simulink model "ModeAdjust"  (R2018b)
settings: Solver=FixedStepDiscrete  StartTime=0.0  StopTime=inf  FixedStep=0.01  RelTol=1e-3
undefined symbols (not defined in the file or in its folder): IfKeSMSbSeatMovBkRclnEnable_Val, IfKeSMSbSeatMovFrwdBkwdEnable_Val, IfKeSMSbSeatMovFtrstEnable_Val, IfKeSMSbSeatMovHdrstFrwdBkwdEnable_Val, IfKeSMSbSeatMovHdUpwdDnwdEnable_Val, IfKeSMSbSeatMovLgrstEnable_Val, IfKeSMSbSeatMovLtwdRtwdEnable_Val, IfVeSMSeStNumConfig, KeSMSbArmscreenMovEnable_Val, KeSMSbSeatMovLgrstExpdEnable_Val, KeSMSuFirstRwStBackPosDelta_Val, KeSMSuFirstRwStBackPosTolr_Val, KeSMSuFirstRwStCushFrntPosDelta_Val, KeSMSuFirstRwStCushFrntPosTolr_Val, KeSMSuFirstRwStCushRePosDelta_Val, KeSMSuFirstRwStCushRePosTolr_Val, KeSMSuFirstRwStFootrestPosDelta_Val, KeSMSuFirstRwStFootrestPosTolr_Val, KeSMSuFirstRwStFwdBkwdPosDelta_Val, KeSMSuFirstRwStFwdBkwdPosTolr_Val, KeSMSuMdMotFinshdTm_Val, KeSMSuMdRetryTm1_Val, KeSMSuModeReqDurgTm_Val, KeSMSuSecRwStArmTochPosDelta_Val, KeSMSuSecRwStArmTochPosTolr_Val, KeSMSuSecRwStBackPosDelta_Val, KeSMSuSecRwStBackPosTolr_Val, KeSMSuSecRwStFtrstUpwdDnwdPosDelta_Val, KeSMSuSecRwStFtrstUpwdDnwdPosTolr_Val, KeSMSuSecRwStFwdBkwdPosDelta_Val, KeSMSuSecRwStFwdBkwdPosTolr_Val, KeSMSuSecRwStHeadrestFwdBkwdPosDelta_Val, KeSMSuSecRwStHeadrestFwdBkwdPosTolr_Val, KeSMSuSecRwStHeadrestUpwdDwnwdPosDelta_Val, KeSMSuSecRwStHeadrestUpwdDwnwdPosTolr_Val, KeSMSuSecRwStLegrestInOutPosDelta_Val, KeSMSuSecRwStLegrestInOutPosTolr_Val, KeSMSuSecRwStLegrestUpwdDwnwdPosDelta_Val, KeSMSuSecRwStLegrestUpwdDwnwdPosTolr_Val, KeSMSuSecRwStLwdRwdPosDelta_Val, KeSMSuSecRwStLwdRwdPosTolr_Val, KeSMSuSecRwStVIPFtrstRefAngle_Val, KeSMSuThirdRwStFwdBkwdPosDelta_Val, KeSMSuThirdRwStFwdBkwdPosTolr_Val, KeSMSuThrdRwCushFoldPosDelta_Val, KeSMSuThrdRwCushFoldPosTolr_Val, KeSMSuThrdRwStBackPosDelta_Val, KeSMSuThrdRwStBackPosTolr_Val, KeSMSw4SLegrstCloseMdSecRwLtStFtrstUpwdDnwdPos_Val, KeSMSw4SLegrstCloseMdSecRwLtStFtrstUpwdDnwdPosMax_Val, KeSMSw4SLegrstCloseMdSecRwLtStFtrstUpwdDnwdPosMin_Val, KeSMSw4SLegrstCloseMdSecRwLtStLgrstOtwdInwdPos_Val, KeSMSw4SLegrstCloseMdSecRwLtStLgrstOtwdInwdPosMax_Val, KeSMSw4SLegrstCloseMdSecRwLtStLgrstOtwdInwdPosMin_Val, KeSMSw4SLegrstCloseMdSecRwLtStLgrstUpwdDnwdPos_Val, KeSMSw4SLegrstCloseMdSecRwLtStLgrstUpwdDnwdPosMax_Val, KeSMSw4SLegrstCloseMdSecRwLtStLgrstUpwdDnwdPosMin_Val, KeSMSw4SLegrstCloseMdSecRwRtStFtrstUpwdDnwdPos_Val, KeSMSw4SLegrstCloseMdSecRwRtStFtrstUpwdDnwdPosMax_Val, KeSMSw4SLegrstCloseMdSecRwRtStFtrstUpwdDnwdPosMin_Val ... (+1138)
libraries: Lib x401
(part 11 of 35)

== system ModeAdjust/ModeAdjustRunnable_sys/ModeAdjust/VIPR4s ==
  SecRwLtStsPoss : Inport
  SecRwLtStPossV : Inport  Port=2
  SecRwRtStChldLkRsp_L : Inport  Port=3
  Recovery_Mod_Left : Inport  Port=4
  ModeStCalib : Inport  Port=5
  StConfig : Inport  Port=6
  SecRwLtStsPoss4s : Inport  Port=7
  SecRwLtStPossV4s : Inport  Port=8
  StConfig4s : Inport  Port=9
  isRtVipArrivedAtTargetPos : Inport  Port=10
  Calib_VIP4sRAdpt : Inport  Port=11
  Enable : EnablePort  StatesWhenEnabling=reset
  Bus Creator1 : BusCreator  Inputs=2
  Bus Selector : BusSelector  OutputSignals=Calib_Drv,Calib_Pass,Calib_2L,Calib_2R,Calib_3L,Calib_3R,Calib_2L4s,Calib_2R4s
  Bus Selector1 : BusSelector  OutputSignals=DrvStConfig,PassStConfig,SecRwLtStConfig,SecRwRtStConfig,ThdRwLtStConfig,ThdRwRtStConfig
  Bus Selector2 : BusSelector  OutputSignals=SecRwLtStConfig,SecRwRtStConfig
  Bus Selector3 : BusSelector  OutputSignals=IfVeSMSuSecRwRtStBkReclnUpwdDnwdPos_Val_read,IfVeSMSuSecRwRtStFrwdBkwdPos_Val_read,IfVeSMSuSecRwRtStHPassStUpwdDnwdPos_Val_read,IfVeSMSuSecRwRtStLgrstUpwdDnwdPos_Val_read,IfVeSMSuSecRwRtStLtwdRtwdPos_Val_read,SecRwRtStArmScrnPos_Val_read
  Bus Selector4 : BusSelector  OutputSignals=IfVeSMSuSecRwRtStBkReclnUpwdDnwdPosV_Val_read,IfVeSMSuSecRwRtStFrwdBkwdPosV_Val_read,IfVeSMSuSecRwRtStHPassStUpwdDnwdPosV_Val_read,IfVeSMSuSecRwRtStLgrstUpwdDnwdPosV_Val_read,IfVeSMSuSecRwRtStLtwdRtwdPosV_Val_read,SecRwRtStArmScrnPosV_Val_read
  Bus Selector5 : BusSelector  OutputSignals=IfVeSMSuSecRwRtStLgrstOtwdInwdPos_Val_read,IfVeSMSuRrRtStFtUpwdDnwdPos_Val_read,IfVeSMSuSecRwRtStHdrstFrwdBkwdPos_Val_read
  Bus Selector6 : BusSelector  OutputSignals=IfVeSMSuSecRwRtStLgrstOtwdInwdPosV_Val_read,IfVeSMSuRrRtStFtUpwdDnwdPosV_Val_read
  Bus Selector7 : BusSelector  OutputSignals=VipRSecRwRtSt.HdrstFrwdBkwdnwdPos,VipRSecRwRtSt.FtrstUpwdDnwdPos
  Chart : Stateflow chart  TreatAsAtomicUnit=on
  Chart1 : Stateflow chart  TreatAsAtomicUnit=on
  Logical Operator : Logic  Inputs=4  AllPortsSameDT=off  OutDataTypeStr=boolean
  Logical Operator1 : Logic  Inputs=3  AllPortsSameDT=off  OutDataTypeStr=boolean
  Logical Operator2 : Logic  AllPortsSameDT=off  OutDataTypeStr=boolean
  Logical Operator3 : Logic  AllPortsSameDT=off  OutDataTypeStr=boolean
  Logical Operator4 : Logic  Operator=NOT  AllPortsSameDT=off  OutDataTypeStr=boolean
  Logical Operator5 : Logic  AllPortsSameDT=off  OutDataTypeStr=boolean
  Logical Operator{6..9} (4 alike) : Logic  Operator=OR  AllPortsSameDT=off  OutDataTypeStr=boolean
  PA_KeSMSw4SSecRwRtStLgrstUpwdDnwdOpenPos1_Val : Constant  Value=KeSMSw4SSecRwRtStLgrstUpwdDnwdOpenPos1_Val
  R2Lt : Subsystem
  Relational Operator : RelationalOperator  OutDataTypeStr=boolean  RndMeth=Simplest
  Relational Operator1 : RelationalOperator  Operator=<  OutDataTypeStr=boolean  RndMeth=Simplest
  Relational Operator2 : RelationalOperator  Operator=<  OutDataTypeStr=boolean  RndMeth=Simplest
  Unit Delay1 : UnitDelay  SampleTime=-1
  Unit Delay3 : UnitDelay  SampleTime=-1
  Unit Delay4 : UnitDelay  SampleTime=-1
  VIP_TrigJudg : Lib/VIP_TrigJudg  SystemSampleTime=-1
  R2Lt_TrgtPoss : Outport  VectorParamsAs1DForOutWhenUnconnected=on
  IfVeSMSuSecRwLtStRclCmdSrv_Val_writeRec : Outport  Port=2
  isAcsMdFeedBackNew_LyL : Outport  Port=3
  R2Lt_TrgtPoss_2 : Outport  Port=4  VectorParamsAs1DForOutWhenUnconnected=on
  wires:
  Unit Delay4/1 -> Logical Operator3/2
  Relational Operator/1 -> Unit Delay3/1
  [lgrstStep2_done] -> Logical Operator2/2
  Logical Operator2/1 -> Unit Delay1/1
  [SecRwLtStLgrstUpwdDnwdPos] -> Relational Operator/1
  [lgrstStep3_done] -> Logical Operator3/1
  Unit Delay3/1 -> Logical Operator2/1
  [lgrstStep2_Chk] -> Unit Delay4/1
  [OpenPos1] -> Relational Operator/2
  R2Lt/4(IfVeSMSuSecRwLtStRclCmdSrv_Val_writeRaw) -> [IfVeSMSuSecRwLtStRclCmdSrv_Val_writeRaw]
  [IfVeSMSuSecRwLtStRclCmdSrv_Val_writeRaw] -> Chart1/2(IfVeSMSuSecRwLtStRclCmdSrv_Val_writeRaw)
  Recovery_Mod_Left/1 -> [Recovery_Mod_Left]
  R2Lt/1(R2Lt_BkHd_Ini) -> [R2LtST_BkHd_ini]
  [Step1_En] -> R2Lt/2(Step1En)
  VIP_TrigJudg/1 -> [EZE_TrigL]
  [EZE_TrigL] -> R2Lt/1(Mode_Trig)
  R2Lt/3(R2Lt_TrgtPoss) -> R2Lt_TrgtPoss/1
  SecRwLtStsPoss/1 -> [Pos], R2Lt/3(SecRwLtStsPoss)
  SecRwLtStPossV/1 -> [PosV], R2Lt/4(SecRwLtStPossV)
  SecRwRtStChldLkRsp_L/1 -> R2Lt/5(SecRwRtStChldLkRsp_L)
  R2Lt/2(R2Lt_BkHd_done) -> [R2LtST_BkHd_done]
  [R2LtST_BkHd_ini] -> Chart/1(R2Lt_ini)
  [R2LtST_BkHd_done] -> Chart/2(R2Lt_done)
  [Recv_L_DoneOK] -> Chart1/3(Md_L_DoneOkRaw)
  [Recv_L_DoneFailed] -> Chart1/4(Md_L_DoneFailedRaw)
  Chart1/2(Md_L_DoneOk) -> [Ly_L_DoneOK]
  Chart1/3(Md_L_DoneFailed) -> [Ly_L_DoneFailed]
  Chart1/1(IfVeSMSuSecRwLtStRclCmdSrv_Val_write) -> IfVeSMSuSecRwLtStRclCmdSrv_Val_writeRec/1  "IfVeSMSuSecRwLtStRclCmdSrv_Val_write"
  Bus Selector/2 -> [ModeStCalib_Pass]  "<Calib_Pass>"
  Bus Selector/5 -> [ModeStCalib_3L]  "<Calib_3L>"
  Bus Selector/3 -> [ModeStCalib_2L]  "<Calib_2L>"
  Bus Selector/1 -> [ModeStCalib_Drv]  "<Calib_Drv>"
  Bus Selector/6 -> [ModeStCalib_3R]  "<Calib_3R>"
  Bus Selector/4 -> [ModeStCalib_2R]  "<Calib_2R>"
  ModeStCalib/1 -> Bus Selector/1
  [ModeStCalib_2R4s] -> R2Lt/6(ModeStCalib_2L)
  [Recovery_Mod_Left] -> VIP_TrigJudg/1
  Bus Creator1/1 -> isAcsMdFeedBackNew_LyL/1
  [Ly_L_DoneOK] -> Bus Creator1/1  "isRtVipDoneOK"
  [Ly_L_DoneFailed] -> Bus Creator1/2  "isRtVipDoneFailed"
  Bus Selector1/6 -> [ThdRwRtStConfig]  "<ThdRwRtStConfig>"
  Bus Selector1/1 -> [DrvStConfig]  "<DrvStConfig>"
  Bus Selector1/3 -> [SecRwLtStConfig]  "<SecRwLtStConfig>"
  Bus Selector1/4 -> [SecRwRtStConfig]  "<SecRwRtStConfig>"
  StConfig/1 -> Bus Selector1/1
  Bus Selector1/2 -> [PassStConfig]  "<PassStConfig>"
  Bus Selector1/5 -> [ThdRwLtStConfig]  "<ThdRwLtStConfig>"
  [SecRwLtStConfig] -> R2Lt/7(StConfig)
  Bus Selector/8 -> [ModeStCalib_2R4s]  "<Calib_2R4s>"
  Bus Selector/7 -> [ModeStCalib_2L4s]  "<Calib_2L4s>"
  SecRwLtStsPoss4s/1 -> [Pos4s], R2Lt/8(SecRwLtStsPoss4s)
  SecRwLtStPossV4s/1 -> [PosV4s], R2Lt/9(SecRwLtStPossV4s)
  StConfig4s/1 -> Bus Selector2/1
  Bus Selector2/1 -> [SecRwLtStConfig4s]  "<SecRwLtStConfig>"
  Bus Selector2/2 -> [SecRwRtStConfig4s]  "<SecRwRtStConfig>"
  [SecRwLtStConfig4s] -> R2Lt/10(StConfig4s)
  [PosV] -> Bus Selector4/1
  Bus Selector4/6 -> [R2LtStArmScrnPosV]  "<SecRwRtStArmScrnPosV_Val_read>"
  Bus Selector3/6 -> [R2LtStArmScrnPos]  "<SecRwRtStArmScrnPos_Val_read>"
  Bus Selector4/5 -> [SecRwLtStLtwdRtwdPosV]  "<IfVeSMSuSecRwRtStLtwdRtwdPosV_Val_read>"
  Bus Selector3/4 -> [SecRwLtStLgrstUpwdDnwdPos]  "<IfVeSMSuSecRwRtStLgrstUpwdDnwdPos_Val_read>"
  Bus Selector3/1 -> [SecRwLtStBkReclnUpwdDnwdPos]  "<IfVeSMSuSecRwRtStBkReclnUpwdDnwdPos_Val_read>"
  Bus Selector3/2 -> [SecRwLtStFrwdBkwdPos]  "<IfVeSMSuSecRwRtStFrwdBkwdPos_Val_read>"
  Bus Selector4/2 -> [SecRwLtStFrwdBkwdPosV]  "<IfVeSMSuSecRwRtStFrwdBkwdPosV_Val_read>"
  Bus Selector4/4 -> [SecRwLtStLgrstUpwdDnwdPosV]  "<IfVeSMSuSecRwRtStLgrstUpwdDnwdPosV_Val_read>"
  Bus Selector3/3 -> [SecRwLtStHPassStUpwdDnwdPos]  "<IfVeSMSuSecRwRtStHPassStUpwdDnwdPos_Val_read>"
  [Pos] -> Bus Selector3/1
  Bus Selector3/5 -> [SecRwLtStLtwdRtwdPos]  "<IfVeSMSuSecRwRtStLtwdRtwdPos_Val_read>"
  Bus Selector4/3 -> [SecRwLtStHPassStUpwdDnwdPosV]  "<IfVeSMSuSecRwRtStHPassStUpwdDnwdPosV_Val_read>"
  Bus Selector4/1 -> [SecRwLtStBkReclnUpwdDnwdPosV]  "<IfVeSMSuSecRwRtStBkReclnUpwdDnwdPosV_Val_read>"
  Bus Selector6/1 -> [SecRwLtStLgrstOtwdInwdPosV]  "<IfVeSMSuSecRwRtStLgrstOtwdInwdPosV_Val_read>"
  [Pos4s] -> Bus Selector5/1
  Bus Selector6/2 -> [RrLtStFtUpwdDnwdPosV]  "<IfVeSMSuRrRtStFtUpwdDnwdPosV_Val_read>"
  [PosV4s] -> Bus Selector6/1
  Bus Selector5/1 -> [SecRwLtStLgrstOtwdInwdPos]  "<IfVeSMSuSecRwRtStLgrstOtwdInwdPos_Val_read>"
  Bus Selector5/2 -> [RrLtStFtUpwdDnwdPos]  "<IfVeSMSuRrRtStFtUpwdDnwdPos_Val_read>"
  [SecRwLtStLgrstUpwdDnwdPos] -> Chart/3(pos)
  [StepEn_LgrstStep1] -> R2Lt/11(StepEn_LgrstStep1)
  [StepEn_LgrstStep2] -> R2Lt/12(StepEn_LgrstStep2)
  [StepEn_LgrstStep3] -> R2Lt/13(StepEn_LgrstStep3)
  R2Lt/5(lgrstStep1_ini) -> [lgrstStep1_ini]
  R2Lt/7(lgrstStep3_ini) -> [lgrstStep3_ini]
  R2Lt/6(lgrstStep2_ini) -> [lgrstStep2_ini]
  R2Lt/8(lgrstStep1_done) -> [lgrstStep1_done]
  R2Lt/10(lgrstStep3_done) -> [lgrstStep3_done]
  R2Lt/9(lgrstStep2_done) -> [lgrstStep2_done]
  [lgrstStep1_done] -> Chart/5(Step1done)
  [lgrstStep1_ini] -> Chart/8(Step1_ini)
  [lgrstStep2_ini] -> Chart/9(Step2_ini)
  [lgrstStep3_ini] -> Chart/10(Step3_ini)
  PA_KeSMSw4SSecRwRtStLgrstUpwdDnwdOpenPos1_Val/1 -> [OpenPos1]
  [OpenPos1] -> Chart/4(openpos1)
  Logical Operator3/1 -> Chart/7(Step3done), [lgrstStep3_Chk]
  Unit Delay1/1 -> Chart/6(Step2done), [lgrstStep2_Chk]
  R2Lt/11(R2Lt_TrgtPoss_2) -> R2Lt_TrgtPoss_2/1
  Logical Operator4/1 -> [Recv_L_DoneFailed]
  isRtVipArrivedAtTargetPos/1 -> [Recv_L_DoneOK], Logical Operator4/1
  [HdUp_Done] -> Logical Operator/3
  [HFwd_Done] -> Logical Operator/4
  [failflg] -> Logical Operator6/2
  Logical Operator1/1 -> Logical Operator6/1
  [R2LtST_BkHd_done] -> Logical Operator/2
  Logical Operator/1 -> Chart1/1(Left_Done)
  Logical Operator6/1 -> Logical Operator/1
  Chart/1(R2Lt_En) -> [Step1_En]
  [HdUp_Done] -> Chart/12(HdUp_Done)
  Chart/7(failflg) -> [failflg]
  Chart/5(HdUp_En) -> [HdUp_En]
  [HFwd_Done] -> Chart/13(HdFwd_Done)
  Chart/2(StepEn_LgrstStep1) -> [StepEn_LgrstStep1]
  Bus Selector7/1 -> Relational Operator1/2  "<HdrstFrwdBkwdnwdPos>"
  [SecRwLtStHdrstFrwdBkwdPos] -> Relational Operator1/1
  Logical Operator5/1 -> Chart/11(chkhdflg)
  Chart/6(HdFwd_En) -> [HdFwd_En]
  Relational Operator1/1 -> Logical Operator5/1
  [ModeStCalib_2R4s] -> Bus Selector7/1
  [SecRwLtStHPassStUpwdDnwdPos] -> Relational Operator2/1
  Bus Selector7/2 -> Relational Operator2/2  "<FtrstUpwdDnwdPos>"
  Chart/4(StepEn_LgrstStep3) -> [StepEn_LgrstStep3]
  Relational Operator2/1 -> Logical Operator5/2
  Chart/3(StepEn_LgrstStep2) -> [StepEn_LgrstStep2]
  R2Lt/14(R2Lt_HdFwd_Ini) -> [HFwd_ini]
  R2Lt/13(R2Lt_HdUp_Done) -> [HdUp_Done]
  R2Lt/15(R2Lt_HdFwd_Done) -> [HFwd_Done]
  R2Lt/12(R2Lt_HdUp_Ini) -> [HdUp_ini]
  [HdFwd_En] -> R2Lt/15(HdFwd_En)
  [HdUp_En] -> R2Lt/14(HdUp_En)
  Bus Selector5/3 -> [SecRwLtStHdrstFrwdBkwdPos]  "<IfVeSMSuSecRwRtStHdrstFrwdBkwdPos_Val_read>"
  Logical Operator7/1 -> Logical Operator1/1
  Logical Operator8/1 -> Logical Operator1/2
  Logical Operator9/1 -> Logical Operator1/3
  [lgrstStep3_Chk] -> Logical Operator9/1
  [lgrstStep2_Chk] -> Logical Operator8/1
  [lgrstStep1_done] -> Logical Operator7/1
  [lgrstStep1_ini] -> Logical Operator7/2
  [lgrstStep2_ini] -> Logical Operator8/2
  [lgrstStep3_ini] -> Logical Operator9/2
  [HdUp_ini] -> Chart/14(HdUp_ini)
  [HFwd_ini] -> Chart/15(HdFwd_ini)
  Calib_VIP4sRAdpt/1 -> R2Lt/16(Calib_VIP4sRAdpt)

== system ModeAdjust/ModeAdjustRunnable_sys/ModeAdjust/AcsMdEntry/Drv ==
  Mode_Trig : Inport
  Step1En : Inport  Port=2
  DrvCurPos : Inport  Port=3
  DrvCurPosV : Inport  Port=4
  ModeStCalib_Drv : Inport  Port=5
  StConfig : Inport  Port=6
  Bus Creator : BusCreator  Inputs=8  OutDataTypeStr=Bus: DrvSeatPos
  Bus Selector : BusSelector  OutputSignals=IfVeSMSuDrvStFtUpwdDnwdPos_Val_read,IfVeSMSuDrvStBkReclnUpwdDnwdPos_Val_read,IfVeSMSuDrvStCshnFrntUpwdDnwdPos_Val_read,IfVeSMSuDrvStCshnRrUpwdDnwdPos_Val_read,IfVeSMSuDrvStFrwdBkwdPos_Val_read
  Bus Selector1 : BusSelector  OutputSignals=IfVeSMSuDrvStFtUpwdDnwdPosV_Val_read,IfVeSMSuDrvStBkReclnUpwdDnwdPosV_Val_read,IfVeSMSuDrvStCshnFrntUpwdDnwdPosV_Val_read,IfVeSMSuDrvStCshnRrUpwdDnwdPosV_Val_read,IfVeSMSuDrvStFrwdBkwdPosV_Val_read
  Bus Selector2 : BusSelector  OutputSignals=BkReclnUpwdDnwdPos,BkReclnUpwdDnwdPosMax,BkReclnUpwdDnwdPosMin,FrwdBkwdPos,FrwdBkwdPosMax,FrwdBkwdPosMin,FtUpwdDnwdPos,FtUpwdDnwdPosMax,FtUpwdDnwdPosMin
  Bus Selector3 : BusSelector  OutputSignals=AcsEntryDrvSt
  Bus Selector4 : BusSelector  OutputSignals=BkReclnUpwdDnwdMovConfig,FrwdBkwdMovConfig,FtUpwdDnwdMovConfig
  DrvSt_DrvStFtUpwdDnwd_Step1 : Lib/CommonUsed  SystemSampleTime=-1
  PA_KeSMSuFirstRwStBackPosDelta_Val : Constant  Value=KeSMSuFirstRwStBackPosDelta_Val
  PA_KeSMSuFirstRwStFootrestPosDelta_Val : Constant  Value=KeSMSuFirstRwStFootrestPosDelta_Val
  PA_KeSMSuFirstRwStFwdBkwdPosDelta_Val : Constant  Value=KeSMSuFirstRwStFwdBkwdPosDelta_Val
  PA_KeSMSuMdMotFinshdTm_Val : Constant  Value=KeSMSuMdMotFinshdTm_Val
  PA_KeSMSuMdRetryTm1_Val : Constant  Value=KeSMSuMdRetryTm1_Val
  PA_KeSMSuModeReqDurgTm_Val : Constant  Value=KeSMSuModeReqDurgTm_Val
  PA_KeSMSwDltTrgtPos_Val{1..3,10,13..16} (8 alike) : Constant  Value=KeSMSwPosInvalidVal_Val
  PA_KeSMSwDltTrgtPos_Val11 : Constant  Value=0  OutDataTypeStr=boolean
  PA_KeSMSwDltTrgtPos_Val5 : Constant  Value=0  OutDataTypeStr=boolean
  DrvSt_Step1_ini : Outport
  DrvSt_Step1_done : Outport  Port=2
  EZE_DrvStTrgtPoss : Outport  Port=3  VectorParamsAs1DForOutWhenUnconnected=on
  wires:
  DrvSt_DrvStFtUpwdDnwd_Step1/4 -> [Step1done_2]
  DrvSt_DrvStFtUpwdDnwd_Step1/3 -> [DrvSt_FtUpwdDnwd_TarPos]
  DrvSt_DrvStFtUpwdDnwd_Step1/2 -> [Step1_2_ArrivedTarPos]
  DrvSt_DrvStFtUpwdDnwd_Step1/1 -> [FtUpwdDnwd_Step1_ini]
  [Tick] -> DrvSt_DrvStFtUpwdDnwd_Step1/11
  PA_KeSMSwDltTrgtPos_Val1/1 -> DrvSt_DrvStFtUpwdDnwd_Step1/10
  PA_KeSMSwDltTrgtPos_Val11/1 -> DrvSt_DrvStFtUpwdDnwd_Step1/9
  [DrvStFtUpwdDnwdPosV] -> DrvSt_DrvStFtUpwdDnwd_Step1/8
  [KeSMSuFirstRwStFootrestPosDelta_Val] -> DrvSt_DrvStFtUpwdDnwd_Step1/7
  [DrvStFtUpwdDnwdPos] -> DrvSt_DrvStFtUpwdDnwd_Step1/3
  [K_DrvStFtUpwdDnwdPos] -> DrvSt_DrvStFtUpwdDnwd_Step1/6
  [K_DrvStFtUpwdDnwdPosMax] -> DrvSt_DrvStFtUpwdDnwd_Step1/5
  [K_DrvStFtUpwdDnwdPosMin] -> DrvSt_DrvStFtUpwdDnwd_Step1/4
  [Step1En] -> DrvSt_DrvStFtUpwdDnwd_Step1/2
  [Trig] -> DrvSt_DrvStFtUpwdDnwd_Step1/1
  PA_KeSMSuModeReqDurgTm_Val/1 -> [Tick]
  Step1En/1 -> [Step1En]
  Mode_Trig/1 -> [Trig]
  Bus Selector1/1 -> [DrvStFtUpwdDnwdPosV]  "<IfVeSMSuDrvStFtUpwdDnwdPosV_Val_read>"
  Bus Selector/4 -> [DrvStCshnRrUpwdDnwdPos]  "<IfVeSMSuDrvStCshnRrUpwdDnwdPos_Val_read>"
  Bus Selector1/2 -> [DrvStBkReclnUpwdDnwdPosV]  "<IfVeSMSuDrvStBkReclnUpwdDnwdPosV_Val_read>"
  Bus Selector/2 -> [DrvStBkReclnUpwdDnwdPos]  "<IfVeSMSuDrvStBkReclnUpwdDnwdPos_Val_read>"
  Bus Selector/1 -> [DrvStFtUpwdDnwdPos]  "<IfVeSMSuDrvStFtUpwdDnwdPos_Val_read>"
  Bus Selector1/4 -> [DrvStCshnRrUpwdDnwdPosV]  "<IfVeSMSuDrvStCshnRrUpwdDnwdPosV_Val_read>"
  Bus Selector1/3 -> [DrvStCshnFrntUpwdDnwdPosV]  "<IfVeSMSuDrvStCshnFrntUpwdDnwdPosV_Val_read>"
  DrvCurPosV/1 -> Bus Selector1/1
  Bus Selector1/5 -> [DrvStFrwdBkwdPosV]  "<IfVeSMSuDrvStFrwdBkwdPosV_Val_read>"
  DrvCurPos/1 -> Bus Selector/1
  Bus Selector/3 -> [DrvStCshnFrntUpwdDnwdPos]  "<IfVeSMSuDrvStCshnFrntUpwdDnwdPos_Val_read>"
  Bus Selector/5 -> [DrvStFrwdBkwdPos]  "<IfVeSMSuDrvStFrwdBkwdPos_Val_read>"
  [Step1done_2] -> DrvSt_Step1_done/1
  [FtUpwdDnwd_Step1_ini] -> DrvSt_Step1_ini/1
  PA_KeSMSwDltTrgtPos_Val14/1 -> Bus Creator/4  "DrvStLgrstUpwdDnwdTrgtPos"
  PA_KeSMSwDltTrgtPos_Val2/1 -> Bus Creator/5  "DrvStBkReclnUpwdDnwdTrgtPos"
  PA_KeSMSwDltTrgtPos_Val10/1 -> Bus Creator/1  "DrvStBlstOtwdInwdTrgtPos"
  PA_KeSMSwDltTrgtPos_Val16/1 -> Bus Creator/7  "DrvStCshnRrUpwdDnwdTrgtPos"
  PA_KeSMSwDltTrgtPos_Val13/1 -> Bus Creator/3  "DrvStHdrstUpwdDnwdTrgtPos"
  [DrvSt_FtUpwdDnwd_TarPos] -> Bus Creator/2  "DrvStFtUpwdDnwdTrgtPos"
  Bus Creator/1 -> EZE_DrvStTrgtPoss/1
  PA_KeSMSwDltTrgtPos_Val15/1 -> Bus Creator/6  "DrvStCshnFrntUpwdDnwdTrgtPos"
  PA_KeSMSwDltTrgtPos_Val3/1 -> Bus Creator/8  "DrvStFrwdBkwdTrgtPos"
  PA_KeSMSuMdMotFinshdTm_Val/1 -> [KeSMSuMdMotFinshdTm_Val]
  PA_KeSMSuFirstRwStFwdBkwdPosDelta_Val/1 -> [KeSMSuFirstRwStFwdBkwdPosDelta_Val]
  PA_KeSMSuFirstRwStFootrestPosDelta_Val/1 -> [KeSMSuFirstRwStFootrestPosDelta_Val]
  PA_KeSMSuFirstRwStBackPosDelta_Val/1 -> [KeSMSuFirstRwStBackPosDelta_Val]
  [KeSMSuMdMotFinshdTm_Val] -> DrvSt_DrvStFtUpwdDnwd_Step1/12
  Bus Selector2/1 -> [K_DrvStBkReclnUpwdDnwdPos]  "<BkReclnUpwdDnwdPos>"
  Bus Selector2/2 -> [K_DrvStBkReclnUpwdDnwdPosMax]  "<BkReclnUpwdDnwdPosMax>"
  Bus Selector2/3 -> [K_DrvStBkReclnUpwdDnwdPosMin]  "<BkReclnUpwdDnwdPosMin>"
  Bus Selector2/4 -> [K_DrvStFrwdBkwdPos]  "<FrwdBkwdPos>"
  Bus Selector2/5 -> [K_DrvStFrwdBkwdPosMax]  "<FrwdBkwdPosMax>"
  Bus Selector2/6 -> [K_DrvStFrwdBkwdPosMin]  "<FrwdBkwdPosMin>"
  Bus Selector2/7 -> [K_DrvStFtUpwdDnwdPos]  "<FtUpwdDnwdPos>"
  Bus Selector2/8 -> [K_DrvStFtUpwdDnwdPosMax]  "<FtUpwdDnwdPosMax>"
  Bus Selector2/9 -> [K_DrvStFtUpwdDnwdPosMin]  "<FtUpwdDnwdPosMin>"
  ModeStCalib_Drv/1 -> Bus Selector3/1
  Bus Selector3/1 -> Bus Selector2/1  "<AcsEntryDrvSt>"
  PA_KeSMSwDltTrgtPos_Val5/1 -> DrvSt_DrvStFtUpwdDnwd_Step1/13
  StConfig/1 -> Bus Selector4/1
  Bus Selector4/1 -> [BkReclnUpwdDnwdMovConfig]  "<BkReclnUpwdDnwdMovConfig>"
  Bus Selector4/2 -> [FrwdBkwdMovConfig]  "<FrwdBkwdMovConfig>"
  Bus Selector4/3 -> [FtUpwdDnwdMovConfig]  "<FtUpwdDnwdMovConfig>"
  [FtUpwdDnwdMovConfig] -> DrvSt_DrvStFtUpwdDnwd_Step1/14
  [CntLow] -> DrvSt_DrvStFtUpwdDnwd_Step1/15
  PA_KeSMSuMdRetryTm1_Val/1 -> [CntLow]

== system ModeAdjust/ModeAdjustRunnable_sys/ModeAdjust/AcsMdEntry/Pass ==
  Mode_Trig : Inport
  Step1En : Inport  Port=2
  PassStPoss : Inport  Port=3
  PassStPossV : Inport  Port=4
  ModeStCalib_Pass : Inport  Port=5
  StConfig : Inport  Port=6
  Bus Creator : BusCreator  Inputs=8  OutDataTypeStr=Bus: PasSeatPos
  Bus Selector : BusSelector  OutputSignals=IfVeSMSuPassStBkReclnUpwdDnwdPos_Val_read,IfVeSMSuPassStCshnFrntUpwdDnwdPos_Val_read,IfVeSMSuPassStCshnRrUpwdDnwdPos_Val_read,IfVeSMSuPassStFrwdBkwdPos_Val_read,IfVeSMSuPassStFtUpwdDnwdPos_Val_read
  Bus Selector1 : BusSelector  OutputSignals=IfVeSMSuPassStBkReclnUpwdDnwdPosV_Val_read,IfVeSMSuPassStCshnFrntUpwdDnwdPosV_Val_read,IfVeSMSuPassStCshnRrUpwdDnwdPosV_Val_read,IfVeSMSuPassStFrwdBkwdPosV_Val_read,IfVeSMSuPassStFtUpwdDnwdPosV_Val_read
  Bus Selector2 : BusSelector  OutputSignals=BkReclnUpwdDnwdPos,BkReclnUpwdDnwdPosMax,BkReclnUpwdDnwdPosMin,FrwdBkwdPos,FrwdBkwdPosMax,FrwdBkwdPosMin,FtUpwdDnwdPos,FtUpwdDnwdPosMax,FtUpwdDnwdPosMin
  Bus Selector3 : BusSelector  OutputSignals=AcsEntryPassSt
  Bus Selector4 : BusSelector  OutputSignals=BkReclnUpwdDnwdMovConfig,FrwdBkwdMovConfig,FtUpwdDnwdMovConfig
  PA_KeSMSuFirstRwStBackPosDelta_Val : Constant  Value=KeSMSuFirstRwStBackPosDelta_Val
  PA_KeSMSuFirstRwStFootrestPosDelta_Val : Constant  Value=KeSMSuFirstRwStFootrestPosDelta_Val
  PA_KeSMSuFirstRwStFwdBkwdPosDelta_Val : Constant  Value=KeSMSuFirstRwStFwdBkwdPosDelta_Val
  PA_KeSMSuMdMotFinshdTm_Val : Constant  Value=KeSMSuMdMotFinshdTm_Val
  PA_KeSMSuMdRetryTm1_Val : Constant  Value=KeSMSuMdRetryTm1_Val
  PA_KeSMSuModeReqDurgTm_Val : Constant  Value=KeSMSuModeReqDurgTm_Val
  PA_KeSMSwDltTrgtPos_Val{1..2,12,14..18} (8 alike) : Constant  Value=KeSMSwPosInvalidVal_Val
  PA_KeSMSwDltTrgtPos_Val11 : Constant  Value=0  OutDataTypeStr=boolean
  PA_KeSMSwDltTrgtPos_Val4 : Constant  Value=0  OutDataTypeStr=boolean
  PassStFtUpwdDnwd_Step2 : Lib/CommonUsed  SystemSampleTime=-1
  Pass_Step1_ini : Outport
  Pass_Step1_done : Outport  Port=2
  PassStTrgtPoss : Outport  Port=3  VectorParamsAs1DForOutWhenUnconnected=on
  wires:
  Mode_Trig/1 -> [Trig]
  Step1En/1 -> [Step1En]
  [Trig] -> PassStFtUpwdDnwd_Step2/1
  [Step1En] -> PassStFtUpwdDnwd_Step2/2
  [K_FtUpwdDnwdPosMin] -> PassStFtUpwdDnwd_Step2/4
  [K_FtUpwdDnwdPosMax] -> PassStFtUpwdDnwd_Step2/5
  [K_FtUpwdDnwdPos] -> PassStFtUpwdDnwd_Step2/6
  [PassStFtUpwdDnwdPos] -> PassStFtUpwdDnwd_Step2/3
  [KeSMSuFirstRwStFootrestPosDelta_Val] -> PassStFtUpwdDnwd_Step2/7
  [PassStFtUpwdDnwdPosV] -> PassStFtUpwdDnwd_Step2/8
  PA_KeSMSwDltTrgtPos_Val11/1 -> PassStFtUpwdDnwd_Step2/9
  PA_KeSMSwDltTrgtPos_Val12/1 -> PassStFtUpwdDnwd_Step2/10
  [Tick] -> PassStFtUpwdDnwd_Step2/11
  PassStFtUpwdDnwd_Step2/2 -> [Step1_2_ArrivedTarPos]
  PassStFtUpwdDnwd_Step2/3 -> [PassStFtUpwdDnwd_TarPos]
  PassStFtUpwdDnwd_Step2/4 -> [Step1done_2]
  Bus Selector/2 -> [PassStCshnFrntUpwdDnwdPos]  "<IfVeSMSuPassStCshnFrntUpwdDnwdPos_Val_read>"
  Bus Selector/5 -> [PassStFtUpwdDnwdPos]  "<IfVeSMSuPassStFtUpwdDnwdPos_Val_read>"
  Bus Selector1/3 -> [PassStCshnRrUpwdDnwdPosV]  "<IfVeSMSuPassStCshnRrUpwdDnwdPosV_Val_read>"
  PassStPossV/1 -> Bus Selector1/1
  Bus Selector/3 -> [PassStCshnRrUpwdDnwdPos]  "<IfVeSMSuPassStCshnRrUpwdDnwdPos_Val_read>"
  Bus Selector1/2 -> [PassStCshnFrntUpwdDnwdPosV]  "<IfVeSMSuPassStCshnFrntUpwdDnwdPosV_Val_read>"
  Bus Selector/1 -> [PassStBkReclnUpwdDnwdPos]  "<IfVeSMSuPassStBkReclnUpwdDnwdPos_Val_read>"
  Bus Selector/4 -> [PassStFrwdBkwdPos]  "<IfVeSMSuPassStFrwdBkwdPos_Val_read>"
  Bus Selector1/4 -> [PassStFrwdBkwdPosV]  "<IfVeSMSuPassStFrwdBkwdPosV_Val_read>"
  Bus Selector1/1 -> [PassStBkReclnUpwdDnwdPosV]  "<IfVeSMSuPassStBkReclnUpwdDnwdPosV_Val_read>"
  PassStPoss/1 -> Bus Selector/1
  Bus Selector1/5 -> [PassStFtUpwdDnwdPosV]  "<IfVeSMSuPassStFtUpwdDnwdPosV_Val_read>"
  PassStFtUpwdDnwd_Step2/1 -> [FtUpwdDnwd_Step1_ini]
  [FtUpwdDnwd_Step1_ini] -> Pass_Step1_ini/1
  [Step1done_2] -> Pass_Step1_done/1
  Bus Creator/1 -> PassStTrgtPoss/1
  PA_KeSMSwDltTrgtPos_Val16/1 -> Bus Creator/4  "PassStCshnRrUpwdDnwdTrgtPos"
  PA_KeSMSwDltTrgtPos_Val2/1 -> Bus Creator/5  "PassStFrwdBkwdTrgtPos"
  PA_KeSMSwDltTrgtPos_Val17/1 -> Bus Creator/7  "PassStHdrstUpwdDnwdTrgtPos"
  PA_KeSMSwDltTrgtPos_Val18/1 -> Bus Creator/8  "PassStLgrstUpwdDnwdTrgtPos"
  PA_KeSMSwDltTrgtPos_Val1/1 -> Bus Creator/1  "PassStBkReclnUpwdDnwdTrgtPos"
  PA_KeSMSwDltTrgtPos_Val14/1 -> Bus Creator/2  "PassStBlstOtwdInwdTrgtPos"
  PA_KeSMSwDltTrgtPos_Val15/1 -> Bus Creator/3  "PassStCshnFrntUpwdDnwdTrgtPos"
  [PassStFtUpwdDnwd_TarPos] -> Bus Creator/6  "PassStFtUpwdDnwdTrgtPos"
  PA_KeSMSuMdMotFinshdTm_Val/1 -> [KeSMSuMdMotFinshdTm_Val]
  PA_KeSMSuFirstRwStFwdBkwdPosDelta_Val/1 -> [KeSMSuFirstRwStFwdBkwdPosDelta_Val]
  PA_KeSMSuFirstRwStFootrestPosDelta_Val/1 -> [KeSMSuFirstRwStFootrestPosDelta_Val]
  PA_KeSMSuFirstRwStBackPosDelta_Val/1 -> [KeSMSuFirstRwStBackPosDelta_Val]
  [KeSMSuMdMotFinshdTm_Val] -> PassStFtUpwdDnwd_Step2/12
  PA_KeSMSuModeReqDurgTm_Val/1 -> [Tick]
  Bus Selector2/4 -> [K_FrwdBkwdPos]  "<FrwdBkwdPos>"
  Bus Selector2/5 -> [K_FrwdBkwdPosMax]  "<FrwdBkwdPosMax>"
  Bus Selector2/7 -> [K_FtUpwdDnwdPos]  "<FtUpwdDnwdPos>"
  Bus Selector2/3 -> [K_BkReclnUpwdDnwdPosMin]  "<BkReclnUpwdDnwdPosMin>"
  Bus Selector2/8 -> [K_FtUpwdDnwdPosMax]  "<FtUpwdDnwdPosMax>"
  Bus Selector2/1 -> [K_BkReclnUpwdDnwdPos]  "<BkReclnUpwdDnwdPos>"
  Bus Selector2/9 -> [K_FtUpwdDnwdPosMin]  "<FtUpwdDnwdPosMin>"
  Bus Selector2/6 -> [K_FrwdBkwdPosMin]  "<FrwdBkwdPosMin>"
  Bus Selector3/1 -> Bus Selector2/1  "<AcsEntryPassSt>"
  ModeStCalib_Pass/1 -> Bus Selector3/1
  Bus Selector2/2 -> [K_BkReclnUpwdDnwdPosMax]  "<BkReclnUpwdDnwdPosMax>"
  PA_KeSMSwDltTrgtPos_Val4/1 -> PassStFtUpwdDnwd_Step2/13
  Bus Selector4/1 -> [BkReclnUpwdDnwdMovConfig]  "<BkReclnUpwdDnwdMovConfig>"
  Bus Selector4/3 -> [FtUpwdDnwdMovConfig]  "<FtUpwdDnwdMovConfig>"
  Bus Selector4/2 -> [FrwdBkwdMovConfig]  "<FrwdBkwdMovConfig>"
  StConfig/1 -> Bus Selector4/1
  [FtUpwdDnwdMovConfig] -> PassStFtUpwdDnwd_Step2/14
  [CntLow] -> PassStFtUpwdDnwd_Step2/15
  PA_KeSMSuMdRetryTm1_Val/1 -> [CntLow]

== system ModeAdjust/ModeAdjustRunnable_sys/ModeAdjust/AcsMdEntry/R2Lt ==
  note: 2L 扶手屏位置
  note: %1锁，2未锁
  Mode_Trig : Inport
  Step1En : Inport  Port=2
  Step2En : Inport  Port=3
  SecRwLtStsPoss : Inport  Port=4
  SecRwLtStPossV : Inport  Port=5
  SecRwRtStChldLkRsp_L : Inport  Port=6
  ModeStCalib_2L : Inport  Port=7
  StConfig : Inport  Port=8
  isR2LtSeatOccupied : Inport  Port=9
  AND : Logic  AllPortsSameDT=off  OutDataTypeStr=boolean
  Bus Creator : BusCreator  Inputs=9  OutDataTypeStr=Bus: SecRwLfSeatPos
  Bus Selector : BusSelector  OutputSignals=IfVeSMSuSecRwLtStBkReclnUpwdDnwdPos_Val_read,IfVeSMSuSecRwLtStFrwdBkwdPos_Val_read,IfVeSMSuSecRwLtStHPassStUpwdDnwdPos_Val_read,IfVeSMSuSecRwLtStLgrstUpwdDnwdPos_Val_read,IfVeSMSuSecRwLtStLtwdRtwdPos_Val_read,IfVeSMSuSecRwLtStArmScrnPos_Val_read
  Bus Selector1 : BusSelector  OutputSignals=IfVeSMSuSecRwLtStBkReclnUpwdDnwdPosV_Val_read,IfVeSMSuSecRwLtStFrwdBkwdPosV_Val_read,IfVeSMSuSecRwLtStHPassStUpwdDnwdPosV_Val_read,IfVeSMSuSecRwLtStLgrstUpwdDnwdPosV_Val_read,IfVeSMSuSecRwLtStLtwdRtwdPosV_Val_read,IfVeSMSuSecRwLtStArmScrnPosV_Val_read
  Bus Selector2 : BusSelector  OutputSignals=ArmScrnPos,ArmScrnPosMax,ArmScrnPosMin,BkReclnUpwdDnwdPos,BkReclnUpwdDnwdPosMax,BkReclnUpwdDnwdPosMin,FrwdBkwdPos,FrwdBkwdPosMax,FrwdBkwdPosMin,HdrstUpwdPos,HdrstUpwdPosMax,HdrstUpwdPosMin,LgrstUpwdPos,LgrstUpwdPosMax,LgrstUpwdPosMin,LtwdRtwdPos,LtwdRtwdPosMax,LtwdRtwdPosMin
  Bus Selector3 : BusSelector  OutputSignals=AcsEntrySecRwLtSt
  Bus Selector4 : BusSelector  OutputSignals=BkReclnUpwdDnwdMovConfig,ArmTouchMovConfig,FrwdBkwdMovConfig,LgrstUpwdMovConfig,LtwdRtwdMovConfig
  Logical Operator1 : Logic  Inputs=3  AllPortsSameDT=off  OutDataTypeStr=boolean
  Logical Operator2 : Logic  Inputs=3  AllPortsSameDT=off  OutDataTypeStr=boolean
  Logical Operator3 : Logic  AllPortsSameDT=off  OutDataTypeStr=boolean
  Logical Operator4 : Logic  AllPortsSameDT=off  OutDataTypeStr=boolean
  Logical Operator5 : Logic  Operator=OR  AllPortsSameDT=off  OutDataTypeStr=boolean
  Logical Operator6 : Logic  AllPortsSameDT=off  OutDataTypeStr=boolean
  NOT : Logic  Operator=NOT  AllPortsSameDT=off  OutDataTypeStr=boolean
  PA_KeSMSuMdMotFinshdTm_Val : Constant  Value=KeSMSuMdMotFinshdTm_Val
  PA_KeSMSuMdRetryTm1_Val : Constant  Value=KeSMSuMdRetryTm1_Val
  PA_KeSMSuModeReqDurgTm_Val : Constant  Value=KeSMSuModeReqDurgTm_Val
  PA_KeSMSuSecRwStArmTochPosDelta_Val : Constant  Value=KeSMSuSecRwStArmTochPosDelta_Val
  PA_KeSMSuSecRwStBackPosDelta_Val : Constant  Value=KeSMSuSecRwStBackPosDelta_Val
  PA_KeSMSuSecRwStFwdBkwdPosDelta_Val : Constant  Value=KeSMSuSecRwStFwdBkwdPosDelta_Val
  PA_KeSMSuSecRwStLegrestUpwdDwnwdPosDelta_Val : Constant  Value=KeSMSuSecRwStLegrestUpwdDwnwdPosDelta_Val
  PA_KeSMSuSecRwStLwdRwdPosDelta_Val : Constant  Value=KeSMSuSecRwStLwdRwdPosDelta_Val
  PA_KeSMSwDltTrgtPos_Val{1,4..5,7..8,10..11,16..17} (9 alike) : Constant  Value=0  OutDataTypeStr=boolean
  PA_KeSMSwDltTrgtPos_Val{3,6,12..15,18..21} (10 alike) : Constant  Value=KeSMSwPosInvalidVal_Val
  PA_KeSMSwDltTrgtPos_Val2 : Constant  Value=SeatChldLkSt.ChldLkSt_Unlock
  PA_KeSMSwDltTrgtPos_Val22 : Constant  Value=3  OutDataTypeStr=uint8
  PA_KeSMSwDltTrgtPos_Val23 : Constant  Value=2  OutDataTypeStr=uint8
  PA_KeSMSwSecRwLtStEasyEntryCllsnPt_Val : Constant  Value=KeSMSwSecRwLtStEasyEntryCllsnPt_Val
  R2LtStArmScrnPos_Step1 : Lib/CommonUsed  SystemSampleTime=-1
  R2LtStFrwdBkwd_Step2 : Lib/CommonUsed  SystemSampleTime=-1
  R2LtSt_BkReclnUpwdDnwd_Step1 : Lib/CommonUsed  SystemSampleTime=-1
  R2LtSt_LgrstUpwdPos_Step1 : Lib/CommonUsed  SystemSampleTime=-1
  R2LtSt_LtwdRtwd_Step2 : Lib/CommonUsed  SystemSampleTime=-1
  Relational Operator : RelationalOperator  Operator=~=  OutDataTypeStr=boolean  RndMeth=Simplest
  Relational Operator1 : RelationalOperator  Operator=<=  OutDataTypeStr=boolean  RndMeth=Simplest
  Relational Operator2 : RelationalOperator  Operator=~=  OutDataTypeStr=boolean  RndMeth=Simplest
  Switch : Switch  Criteria=u2 ~= 0
  R2Lt_Step1_Ini : Outport
  R2Lt_Step2_Ini : Outport  Port=2
  R2Lt_Step1_done : Outport  Port=3
  R2Lt_Step2_done : Outport  Port=4
  R2Lt_TrgtPoss : Outport  Port=5  VectorParamsAs1DForOutWhenUnconnected=on
  R2Lt_SpdCtrl : Outport  Port=6
  wires:
  [K_BkReclnUpwdDnwdPosMax] -> R2LtSt_BkReclnUpwdDnwd_Step1/5
  [Trig] -> R2LtSt_BkReclnUpwdDnwd_Step1/1
  Mode_Trig/1 -> [Trig]
  [KeSMSuSecRwStBackPosDelta_Val] -> R2LtSt_BkReclnUpwdDnwd_Step1/7
  [SecRwLtStFrwdBkwdPos] -> R2LtStFrwdBkwd_Step2/3
  [K_FrwdBkwdPosMax] -> R2LtStFrwdBkwd_Step2/5
  [KeSMSuSecRwStFwdBkwdPosDelta_Val] -> R2LtStFrwdBkwd_Step2/7
  [K_FrwdBkwdPosMin] -> R2LtStFrwdBkwd_Step2/4
  R2LtSt_BkReclnUpwdDnwd_Step1/1 -> [ReclnUpwdDnwd_Step1_ini]
  R2LtStFrwdBkwd_Step2/1 -> [FrwdBkwd_inidone_Step2]
  [K_BkReclnUpwdDnwdPosMin] -> R2LtSt_BkReclnUpwdDnwd_Step1/4
  R2LtSt_BkReclnUpwdDnwd_Step1/2 -> [Step1_1_ArrivedTarPos]
  [SecRwLtStBkReclnUpwdDnwdPos] -> R2LtSt_BkReclnUpwdDnwd_Step1/3
  [K_BkReclnUpwdDnwdPos] -> R2LtSt_BkReclnUpwdDnwd_Step1/6
  PA_KeSMSwDltTrgtPos_Val3/1 -> R2LtSt_BkReclnUpwdDnwd_Step1/10
  R2LtSt_BkReclnUpwdDnwd_Step1/3 -> [R2Lt_BkReclnUpwdDnwd_TarPos]
  R2LtSt_BkReclnUpwdDnwd_Step1/4 -> [Step1done_1]
  [Step1En] -> R2LtSt_BkReclnUpwdDnwd_Step1/2
  [Trig] -> R2LtStFrwdBkwd_Step2/1
  [Step2En] -> R2LtStFrwdBkwd_Step2/2
  [K_FrwdBkwdPos] -> R2LtStFrwdBkwd_Step2/6
  [SecRwLtStFrwdBkwdPosV] -> R2LtStFrwdBkwd_Step2/8
  [ChildLocker] -> R2LtSt_BkReclnUpwdDnwd_Step1/9
  PA_KeSMSwDltTrgtPos_Val16/1 -> R2LtStFrwdBkwd_Step2/9
  PA_KeSMSwDltTrgtPos_Val6/1 -> R2LtStFrwdBkwd_Step2/10
  [Tick] -> R2LtSt_BkReclnUpwdDnwd_Step1/11
  [Tick] -> R2LtStFrwdBkwd_Step2/11
  R2LtStFrwdBkwd_Step2/3 -> [R2LtStFrwdBkwd_TarPos]
  R2LtStFrwdBkwd_Step2/4 -> [Step2done_1]
  Bus Selector1/3 -> [SecRwLtStHPassStUpwdDnwdPosV]  "<IfVeSMSuSecRwLtStHPassStUpwdDnwdPosV_Val_read>"
  Bus Selector/5 -> [SecRwLtStLtwdRtwdPos]  "<IfVeSMSuSecRwLtStLtwdRtwdPos_Val_read>"
  SecRwLtStsPoss/1 -> Bus Selector/1
  Bus Selector1/4 -> [SecRwLtStLgrstUpwdDnwdPosV]  "<IfVeSMSuSecRwLtStLgrstUpwdDnwdPosV_Val_read>"
  SecRwLtStPossV/1 -> Bus Selector1/1
  Bus Selector/3 -> [SecRwLtStHPassStUpwdDnwdPos]  "<IfVeSMSuSecRwLtStHPassStUpwdDnwdPos_Val_read>"
  Bus Selector1/5 -> [SecRwLtStLtwdRtwdPosV]  "<IfVeSMSuSecRwLtStLtwdRtwdPosV_Val_read>"
  Bus Selector/4 -> [SecRwLtStLgrstUpwdDnwdPos]  "<IfVeSMSuSecRwLtStLgrstUpwdDnwdPos_Val_read>"
  Bus Selector/2 -> [SecRwLtStFrwdBkwdPos]  "<IfVeSMSuSecRwLtStFrwdBkwdPos_Val_read>"
  Bus Selector1/1 -> [SecRwLtStBkReclnUpwdDnwdPosV]  "<IfVeSMSuSecRwLtStBkReclnUpwdDnwdPosV_Val_read>"
  Bus Selector1/2 -> [SecRwLtStFrwdBkwdPosV]  "<IfVeSMSuSecRwLtStFrwdBkwdPosV_Val_read>"
  Bus Selector/1 -> [SecRwLtStBkReclnUpwdDnwdPos]  "<IfVeSMSuSecRwLtStBkReclnUpwdDnwdPos_Val_read>"
  SecRwRtStChldLkRsp_L/1 -> Relational Operator/1
  PA_KeSMSwDltTrgtPos_Val2/1 -> Relational Operator/2
  Relational Operator/1 -> [ChildLocker]
  [Trig] -> R2LtSt_LgrstUpwdPos_Step1/1
  [Step1En] -> R2LtSt_LgrstUpwdPos_Step1/2
  [K_LgrstUpwdPosMin] -> R2LtSt_LgrstUpwdPos_Step1/4
  [K_LgrstUpwdPosMax] -> R2LtSt_LgrstUpwdPos_Step1/5
  [K_LgrstUpwdPos] -> R2LtSt_LgrstUpwdPos_Step1/6
  [SecRwLtStLgrstUpwdDnwdPos] -> R2LtSt_LgrstUpwdPos_Step1/3
  [SecRwLtStBkReclnUpwdDnwdPosV] -> R2LtSt_BkReclnUpwdDnwd_Step1/8
  [KeSMSuSecRwStLegrestUpwdDwnwdPosDelta_Val] -> R2LtSt_LgrstUpwdPos_Step1/7
  [SecRwLtStLgrstUpwdDnwdPosV] -> R2LtSt_LgrstUpwdPos_Step1/8
  PA_KeSMSwDltTrgtPos_Val11/1 -> R2LtSt_LgrstUpwdPos_Step1/9
  PA_KeSMSwDltTrgtPos_Val12/1 -> R2LtSt_LgrstUpwdPos_Step1/10
  [Tick] -> R2LtSt_LgrstUpwdPos_Step1/11
  R2LtSt_LgrstUpwdPos_Step1/1 -> [LgrstUpwd_Step1_ini]
  R2LtSt_LgrstUpwdPos_Step1/2 -> [Step1_2_ArrivedTarPos]
  R2LtSt_LgrstUpwdPos_Step1/3 -> [R2Lt_LgrstUpwd_TarPos]
  R2LtSt_LgrstUpwdPos_Step1/4 -> [Step1done_2]
  [Trig] -> R2LtStArmScrnPos_Step1/1
  [Step1En] -> R2LtStArmScrnPos_Step1/2
  [IfVeSMSuSecRwLtStArmScrnPos] -> R2LtStArmScrnPos_Step1/3
  PA_KeSMSwDltTrgtPos_Val13/1 -> R2LtStArmScrnPos_Step1/10
  [Tick] -> R2LtStArmScrnPos_Step1/11
  [K_ArmScrnPosMax] -> R2LtStArmScrnPos_Step1/5
  [K_ArmScrnPosMin] -> R2LtStArmScrnPos_Step1/4
  [K_ArmScrnPos] -> R2LtStArmScrnPos_Step1/6
  [KeSMSuSecRwStArmTochPosDelta_Val] -> R2LtStArmScrnPos_Step1/7
  [IfVeSMSuSecRwLtStArmScrnPosV] -> R2LtStArmScrnPos_Step1/8
  PA_KeSMSwDltTrgtPos_Val10/1 -> R2LtStArmScrnPos_Step1/9
  [Step1done_1] -> Logical Operator2/1
  [Step1done_2] -> Logical Operator2/2
  [Step1done_3] -> Logical Operator2/3
  [K_LtwdRtwdPosMax] -> R2LtSt_LtwdRtwd_Step2/5
  [K_LtwdRtwdPos] -> R2LtSt_LtwdRtwd_Step2/6
  [K_LtwdRtwdPosMin] -> R2LtSt_LtwdRtwd_Step2/4
  [SecRwLtStLtwdRtwdPos] -> R2LtSt_LtwdRtwd_Step2/3
  [SecRwLtStLtwdRtwdPosV] -> R2LtSt_LtwdRtwd_Step2/8
  [Trig] -> R2LtSt_LtwdRtwd_Step2/1
  PA_KeSMSwDltTrgtPos_Val14/1 -> R2LtSt_LtwdRtwd_Step2/10
  [Tick] -> R2LtSt_LtwdRtwd_Step2/11
  [KeSMSuSecRwStLwdRwdPosDelta_Val] -> R2LtSt_LtwdRtwd_Step2/7
  PA_KeSMSwDltTrgtPos_Val17/1 -> R2LtSt_LtwdRtwd_Step2/9
  R2LtSt_LtwdRtwd_Step2/4 -> [Step2done_2]
  R2LtSt_LtwdRtwd_Step2/1 -> [LtwdRtwd_inidone_Step2]
  R2LtSt_LtwdRtwd_Step2/3 -> [R2LtSt_LtwdRtwd_TarPos]
  [Step2done_1] -> Logical Operator4/1
  [Step2done_2] -> Logical Operator4/2
  Logical Operator3/1 -> R2LtSt_LtwdRtwd_Step2/2
  [Step2En] -> Logical Operator3/2
  Logical Operator5/1 -> Logical Operator3/1
  [Step2done_1] -> Logical Operator5/1
  [SecRwLtStFrwdBkwdPos] -> Relational Operator1/1
  Relational Operator1/1 -> Logical Operator5/2
  [ReclnUpwdDnwd_Step1_ini] -> Logical Operator1/1
  [LgrstUpwd_Step1_ini] -> Logical Operator1/2
  [ArmScrn_Step1_ini] -> Logical Operator1/3
  Logical Operator1/1 -> R2Lt_Step1_Ini/1
  [FrwdBkwd_inidone_Step2] -> Logical Operator6/1
  [LtwdRtwd_inidone_Step2] -> Logical Operator6/2
  Logical Operator6/1 -> R2Lt_Step2_Ini/1
  Logical Operator2/1 -> R2Lt_Step1_done/1
  Logical Operator4/1 -> R2Lt_Step2_done/1
  R2LtStFrwdBkwd_Step2/2 -> [Step2_1_ArrivedTarPos]
  R2LtSt_LtwdRtwd_Step2/2 -> [Step2_2_ArrivedTarPos]
  PA_KeSMSwDltTrgtPos_Val21/1 -> Bus Creator/6  "SecRwLtStHdrstUpwdDnwdTrgtPos"
  Bus Creator/1 -> R2Lt_TrgtPoss/1
  [R2Lt_LgrstUpwd_TarPos] -> Bus Creator/7  "SecRwLtStLgrstUpwdDnwdTrgtPos"
  PA_KeSMSwDltTrgtPos_Val19/1 -> Bus Creator/3  "SecRwLtStCshnFrntUpwdDnwdTrgtPos"
  [R2LtSt_LtwdRtwd_TarPos] -> Bus Creator/8  "SecRwLtStLtwdRtwdTrgtPos"
  PA_KeSMSwDltTrgtPos_Val18/1 -> Bus Creator/2  "SecRwLtStBlstOtwdInwdTrgtPos"
  [R2Lt_BkReclnUpwdDnwd_TarPos] -> Bus Creator/1  "SecRwLtStBkReclnUpwdDnwdTrgtPos"
  [R2LtStFrwdBkwd_TarPos] -> Bus Creator/5  "SecRwLtStFrwdBkwdTrgtPos"
  PA_KeSMSwDltTrgtPos_Val20/1 -> Bus Creator/4  "SecRwLtStCshnRrUpwdDnwdTrgtPos"
  Step1En/1 -> [Step1En]
  Step2En/1 -> [Step2En]
  R2LtStArmScrnPos_Step1/1 -> [ArmScrn_Step1_ini]
  R2LtStArmScrnPos_Step1/2 -> [Step1_3_ArrivedTarPos]
  R2LtStArmScrnPos_Step1/4 -> [Step1done_3]
  PA_KeSMSuModeReqDurgTm_Val/1 -> [Tick]
  R2LtStArmScrnPos_Step1/3 -> [SecRwLtStArmScrnTrgtPos]
  [SecRwLtStArmScrnTrgtPos] -> Bus Creator/9  "SecRwLtStArmScrnTrgtPos"
  PA_KeSMSuSecRwStFwdBkwdPosDelta_Val/1 -> [KeSMSuSecRwStFwdBkwdPosDelta_Val]
  PA_KeSMSuSecRwStLwdRwdPosDelta_Val/1 -> [KeSMSuSecRwStLwdRwdPosDelta_Val]
  PA_KeSMSuSecRwStLegrestUpwdDwnwdPosDelta_Val/1 -> [KeSMSuSecRwStLegrestUpwdDwnwdPosDelta_Val]
  PA_KeSMSuMdMotFinshdTm_Val/1 -> [KeSMSuMdMotFinshdTm_Val]
  PA_KeSMSuSecRwStBackPosDelta_Val/1 -> [KeSMSuSecRwStBackPosDelta_Val]
  PA_KeSMSuSecRwStArmTochPosDelta_Val/1 -> [KeSMSuSecRwStArmTochPosDelta_Val]
  [KeSMSuMdMotFinshdTm_Val] -> R2LtSt_BkReclnUpwdDnwd_Step1/12
  [KeSMSuMdMotFinshdTm_Val] -> R2LtSt_LgrstUpwdPos_Step1/12
  [KeSMSuMdMotFinshdTm_Val] -> R2LtStArmScrnPos_Step1/12
  [KeSMSuMdMotFinshdTm_Val] -> R2LtSt_LtwdRtwd_Step2/12
  [KeSMSuMdMotFinshdTm_Val] -> R2LtStFrwdBkwd_Step2/12
  Bus Selector/6 -> [IfVeSMSuSecRwLtStArmScrnPos]  "<IfVeSMSuSecRwLtStArmScrnPos_Val_read>"
  Bus Selector1/6 -> [IfVeSMSuSecRwLtStArmScrnPosV]  "<IfVeSMSuSecRwLtStArmScrnPosV_Val_read>"
  PA_KeSMSwSecRwLtStEasyEntryCllsnPt_Val/1 -> Relational Operator1/2
  Bus Selector2/7 -> [K_FrwdBkwdPos]  "<FrwdBkwdPos>"
  Bus Selector2/8 -> [K_FrwdBkwdPosMax]  "<FrwdBkwdPosMax>"
  Bus Selector2/6 -> [K_BkReclnUpwdDnwdPosMin]  "<BkReclnUpwdDnwdPosMin>"
  Bus Selector2/4 -> [K_BkReclnUpwdDnwdPos]  "<BkReclnUpwdDnwdPos>"
  Bus Selector2/9 -> [K_FrwdBkwdPosMin]  "<FrwdBkwdPosMin>"
  Bus Selector3/1 -> Bus Selector2/1  "<AcsEntrySecRwLtSt>"
  ModeStCalib_2L/1 -> Bus Selector3/1
  Bus Selector2/5 -> [K_BkReclnUpwdDnwdPosMax]  "<BkReclnUpwdDnwdPosMax>"
  Bus Selector2/2 -> [K_ArmScrnPosMax]  "<ArmScrnPosMax>"
  Bus Selector2/1 -> [K_ArmScrnPos]  "<ArmScrnPos>"
  Bus Selector2/3 -> [K_ArmScrnPosMin]  "<ArmScrnPosMin>"
  Bus Selector2/10 -> [K_HdrstUpwdPos]  "<HdrstUpwdPos>"
  Bus Selector2/11 -> [K_HdrstUpwdPosMax]  "<HdrstUpwdPosMax>"
  Bus Selector2/12 -> [K_HdrstUpwdPosMin]  "<HdrstUpwdPosMin>"
  Bus Selector2/13 -> [K_LgrstUpwdPos]  "<LgrstUpwdPos>"
  Bus Selector2/14 -> [K_LgrstUpwdPosMax]  "<LgrstUpwdPosMax>"
  Bus Selector2/15 -> [K_LgrstUpwdPosMin]  "<LgrstUpwdPosMin>"
  Bus Selector2/16 -> [K_LtwdRtwdPos]  "<LtwdRtwdPos>"
  Bus Selector2/17 -> [K_LtwdRtwdPosMax]  "<LtwdRtwdPosMax>"
  Bus Selector2/18 -> [K_LtwdRtwdPosMin]  "<LtwdRtwdPosMin>"
  PA_KeSMSwDltTrgtPos_Val1/1 -> R2LtSt_BkReclnUpwdDnwd_Step1/13
  PA_KeSMSwDltTrgtPos_Val4/1 -> R2LtSt_LgrstUpwdPos_Step1/13
  PA_KeSMSwDltTrgtPos_Val5/1 -> R2LtStArmScrnPos_Step1/13
  PA_KeSMSwDltTrgtPos_Val7/1 -> R2LtSt_LtwdRtwd_Step2/13
  PA_KeSMSwDltTrgtPos_Val8/1 -> R2LtStFrwdBkwd_Step2/13
  StConfig/1 -> Bus Selector4/1
  Bus Selector4/4 -> [LgrstUpwdMovConfig]  "<LgrstUpwdMovConfig>"
  Bus Selector4/3 -> [FrwdBkwdMovConfig]  "<FrwdBkwdMovConfig>"
  Bus Selector4/2 -> [ArmTouchMovConfig]  "<ArmTouchMovConfig>"
  Bus Selector4/1 -> [BkReclnUpwdDnwdMovConfig]  "<BkReclnUpwdDnwdMovConfig>"
  Bus Selector4/5 -> [LtwdRtwdMovConfig]  "<LtwdRtwdMovConfig>"
  [ArmTouchMovConfig] -> R2LtStArmScrnPos_Step1/14
  [LgrstUpwdMovConfig] -> R2LtSt_LgrstUpwdPos_Step1/14
  [BkReclnUpwdDnwdMovConfig] -> R2LtSt_BkReclnUpwdDnwd_Step1/14
  [FrwdBkwdMovConfig] -> R2LtStFrwdBkwd_Step2/14
  [LtwdRtwdMovConfig] -> R2LtSt_LtwdRtwd_Step2/14
  [CntLow] -> R2LtStArmScrnPos_Step1/15
  [CntLow] -> R2LtStFrwdBkwd_Step2/15
  [CntLow] -> R2LtSt_BkReclnUpwdDnwd_Step1/15
  [CntLow] -> R2LtSt_LgrstUpwdPos_Step1/15
  [CntLow] -> R2LtSt_LtwdRtwd_Step2/15
  PA_KeSMSuMdRetryTm1_Val/1 -> [CntLow]
  [R2LtStFrwdBkwd_TarPos] -> Relational Operator2/1  "SecRwLtStFrwdBkwdTrgtPos"
  Switch/1 -> R2Lt_SpdCtrl/1
  PA_KeSMSwDltTrgtPos_Val22/1 -> Switch/1
  PA_KeSMSwDltTrgtPos_Val15/1 -> Relational Operator2/2  "SecRwLtStHdrstUpwdDnwdTrgtPos"
  AND/1 -> Switch/2
  isR2LtSeatOccupied/1 -> NOT/1
  NOT/1 -> AND/1
  Relational Operator2/1 -> AND/2
  PA_KeSMSwDltTrgtPos_Val23/1 -> Switch/3
